simulink model "rtlsdr_datafm_ascii_audio"  (R2014b)
settings: Solver=ode45  StartTime=0.0  StopTime=60  RelTol=1e-3
PreLoadFcn:
  | %%%%%%%%%%%%%%%%%%%%%%%%%%%%%%%%%%%%%%%%%%%%%%%%%%%%%%%%%%%%%%%%%%%%%%%%%%%
  | % check to see if Simulink library folder is missing from the MATLAB path %
  | %%%%%%%%%%%%%%%%%%%%%%%%%%%%%%%%%%%%%%%%%%%%%%%%%%%%%%%%%%%%%%%%%%%%%%%%%%%
  | if isempty(strfind(path, 'rtlsdr_book_library'))
  | 
  |     % create error window
  |     fig_error = figure(...
  |         'Name', 'Error: RTL-SDR Book Library',...
  |         'Toolbar','none',...
  |         'MenuBar','none',...
  |         'NumberTitle','off',...
  |         'Resize','off',...
  |         'WindowStyle','modal');
  |     fig_error.Position(3) = 600;
  |     fig_error.Position(4) = 150;
  |     fig_axes = axes(...
  |         'Parent',fig_error,...
  |         'Position',[0,0,1,1],...
  |         'visible','off');
  |     % error message
  |     t_title = text(.05,.8,...
  |         'MISSING DIRECTORIES',...
  |         'FontSize',11.5);
  |     t_body = text(.075,.6,...
  |         [{'Simulink cannot find the  \it{<root>}\rm / \it{rtlsdr\_book\_library}\rm  folder in the \it{MATLAB Path}\rm.'},...
  |         {'Please set the MATLAB path following the instructions given in Exercise 2.4.'}],...
  |         'FontSize',10.5);
  |     % buttons
  |     btn_path = uicontrol(...
  |         'Parent',fig_error,...
  |         'String','Set Path Now',...
  |         'FontSize',10,...
  |         'Callback', 'pathtool; close(fig_error);',...
  |         'Position', [fig_error.Position(3)/2-210, 30, 200, 30]);
  |     btn_abort = uicontrol(...
  |         'Parent',fig_error,...
  |         'String','No thanks',...
  |         'FontSize',10,...
  |         'Callback', 'close(fig_error); abort=1;',...
  |         'Position', [fig_error.Position(3)/2+10, 30, 200, 30]);
  | 
  |     % pause to allow user to interact with error box
  |     uiwait(fig_error);
  | 
  |     % abort simulation
  |     try
  |         if abort==1
  |             set_param(gcs, 'SimulationCommand', 'stop');
  |         end
  |     end
  | 
  |     % if user has set path, allow diagram to be updated
  |     if ~exist('abort','var')
  |         % create error window
  |         fig_update = figure(...
  |             'Name', 'Update Diagram',...
  |             'Toolbar','none',...
  |             'MenuBar','none',...
  |             'NumberTitle','off',...
  |             'Resize','off');
  |         fig_update.Position(3) = 400;
  |         fig_update.Position(4) = 120;
  |         fig_axes = axes(...
  |             'Parent',fig_update,...
  |             'Position',[0,0,1,1],...
  |             'visible','off');
  |         % instruction message
  |         t_body = text(.075,.7,...
  |             'Once you have set the path, update the block diagram',...
  |             'FontSize',10.5);
  |         % button
  |         btn_update = uicontrol(...
  |             'Parent',fig_update,...
  |             'String','Update Block Diagram',...
  |             'FontSize',10,...
  |             'Callback', 'set_param(gcs,''SimulationCommand'',''update''); close(gcf)',...
  |             'Position', [fig_update.Position(3)/2-100, 30, 200, 30]);
  |     end
  | 
  |     % clear error components
  |     clear('fig_error','fig_update','fig_axes','t_title','t_body','btn_path','btn_abort','btn_update','abort');
  | 
  | end
  | %%%%%%%%%%%%%%%%%%%%%%%%%%%%%%%%%%%%%%%%%%%%%%%%%%%%%%%%%%%%%%%%%%%%%%%%%%%
undefined symbols (not defined in the file): dfilt, fdesignblkfcn, gcbh, rec, startfcn_spectrum_analyzer
libraries: simulink x5, dsparch4 x3, rtlsdr_book_library x3, dspmlti4 x2, commutil2 x2, commrfcorlib x1, dspstat3 x1, dspmtrx3 x1, sdrrlib x1, dspsnks4 x1
CloseFcn:
  | closefcn_model;
Description:
  | Software, Simulation Examples and Design Exercises Licence Agreement
  | 
  | This license agreement refers to the simulation examples, design exercises and files,
  | and associated software MATLAB and Simulink resources that accompany the book:
  | 
  |      Title: Software Defined Radio using MATLAB & Simulink and the RTL-SDR
  |      Published by Strathclyde Academic Media, 2015
  |      Authored by Robert W. Stewart, Kenneth W. Barlee, Dale S.W. Atkinson,
  |      and Louise H. Crockett
  | 
  | and made available as a download from, www.desktopSDR.com or variously acquired
  | by other means such as via USB storage, cloud storage, disk or any other electronic
  | or optical or magnetic storage mechanism. These files and associated software may
  | be used subject to the terms of agreement of the conditions below:
  | 
  |     Copyright © 2015 Robert W. Stewart, Kenneth W. Barlee, Dale S.W. Atkinson,
  |     and Louise H. Crockett
  |     All rights reserved.
  | 
  | Redistribution and use in source and binary forms, with or without modification, are
  | permitted provided that the following conditions are met:
  | 
  |    1.  Redistributions of source code must retain the above copyright notice, this list of
  |         conditions and the following disclaimer.
  | 
  |    2.  Redistributions in binary form must reproduce the above copyright notice, this
  |         list of conditions and the following disclaimer in the documentation and/or other
  |         materials provided with the distribution.
  | 
  |    3.  Neither the name of the copyright holder nor the names of its contributors may
  |         be used to endorse or promote products derived from this software without
  |         specific prior written permission.
  | 
  |    4.  In all cases, the software is, and all modifications and derivatives of the
  |         software shall be, licensed to you solely for use in conjunction with The
  |         MathWorks, Inc. products and service offerings.
  | 
  | THIS SOFTWARE IS PROVIDED BY THE COPYRIGHT HOLDERS AND CONTRIBUTORS
  | "AS IS" AND ANY EXPRESS OR IMPLIED WARRANTIES, INCLUDING, BUT NOT LIMITED
  | TO, THE IMPLIED WARRANTIES OF MERCHANTABILITY AND FITNESS FOR A
  | PARTICULAR PURPOSE ARE DISCLAIMED. IN NO EVENT SHALL THE COPYRIGHT
  | HOLDER OR CONTRIBUTORS BE LIABLE FOR ANY DIRECT, INDIRECT, INCIDENTAL,
  | SPECIAL, EXEMPLARY, OR CONSEQUENTIAL DAMAGES (INCLUDING, BUT NOT
  | LIMITED TO, PROCUREMENT OF SUBSTITUTE GOODS OR SERVICES; LOSS OF USE,
  | DATA, OR PROFITS; OR BUSINESS INTERRUPTION) HOWEVER CAUSED AND ON ANY
  | THEORY OF LIABILITY, WHETHER IN CONTRACT, STRICT LIABILITY, OR TORT
  | (INCLUDING NEGLIGENCE OR OTHERWISE) ARISING IN ANY WAY OUT OF THE USE
  | OF THIS SOFTWARE, EVEN IF ADVISED OF THE POSSIBILITY OF SUCH DAMAGE.
  | 
  | 
  | Audio Tracks used in Simulations Examples and Design Exercises
  | 
  | The music and vocal files used within the Examples files and software within the book
  | were variously written, arranged, performed, recorded and produced by Garrey Rice,
  | Adam Struth, Jamie Struth, Iain Thistlethwaite and also Marshall Craigmyle who
  | collectively, and individually where appropriate, assert and retain all of their copyright,
  | performance and artistic rights. Permission to use and reproduce this music is
  | granted for all purposes associated with MATLAB and Simulink software and the
  | simulation examples and design exercises files that accompany this book. Requests to
  | use the music for any other purpose should be directed to: info@desktopSDR.com.
  | For information on music track names, full credits, and links to the musicians please
  | refer to www.desktopSDR.com/more/audio.
settings Model: SimulationMode=accelerator  Creator=desktopSDR Team  LastModifiedBy=desktopSDR Team
settings DataIOCC: LimitDataPoints=off  SaveOutput=off  SignalLogging=off  SaveTime=off

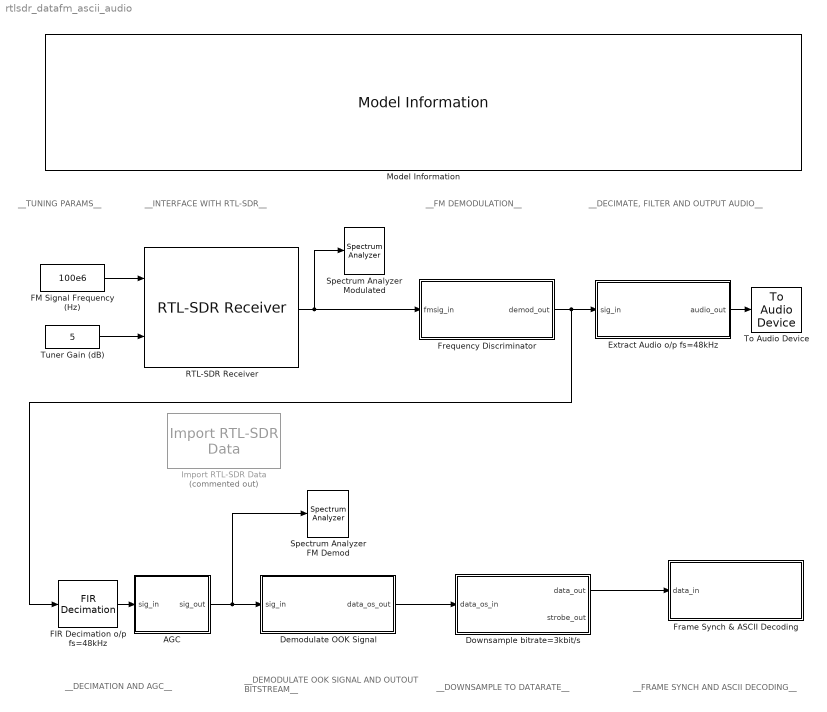
== system rtlsdr_datafm_ascii_audio ==
  note: __FRAME SYNCH AND ASCII DECODING__
  note: __DECIMATION AND AGC__
  note: __DOWNSAMPLE TO DATARATE__
  note: __DEMODULATE OOK SIGNAL
      | AND OUTOUT BITSTREAM__
  note: __FM DEMODULATION__
  note: __INTERFACE WITH RTL-SDR__
  note: __TUNING PARAMS__
  note: __DECIMATE, FILTER AND OUTPUT AUDIO__
  AGC : Subsystem
  Demodulate OOK Signal : Subsystem
  Downsample bitrate=3kbit/s : Subsystem  mask{fs=3e3}
      mask prompts: fs "Data bitrate (bit/s):"
      mask help: This block is used to downsample the received (oversampled) data back to its original bitrate. It comprises of an edge detector and a sampler.
  Extract Audio o/p fs=48kHz : Subsystem
  FIR Decimation o/p fs=48kHz : dspmlti4/FIR Decimation  h=firpm(150, [0 15e3 20e3 (240e3/2)]/(240e3/2), [1 1 0 0], [1 1],20)  D=5  filtStruct=Direct form  framing=Allow multirate processing  inputOffset=0  outputBufInitCond=0  InputProcessing=Columns as channels (frame based)  firstCoeffDataTypeStr=Inherit: Same word length as input  firstCoeffLastDataTypeStr=Inherit: Same word length as input  firstCoeffMin=[]  firstCoeffMax=[]  outputDataTypeStr=Inherit: Same as accumulator  outputLastDataTypeStr=Inherit: Same as accumulator  outputMin=[]  outputMax=[]  roundingMode=Floor  overflowMode=off  FilterSource=Specify via dialog  FilterObject=Hm_firdecim
      settings: allowOverrides=off
  "FM Signal Frequency (Hz) " : Constant  Value=100e6
  Frame Synch & ASCII Decoding : Subsystem  mask(Receiver Parameter Settings){msg_len=32, fs=3e3, ascii_len=8}
      mask prompts: msg_len "Message Length (chars)"; fs "Sampling Frequency"; ascii_len "ACSII Length"
      mask help: The subsystem implements frame synchronisation to re-frame the received data back to its original frame structure. The preamble is then removed before the payload data is ASCII decoded back to the transmitted string.
      mask Callback msg_len: ASCII_receive_mtchd_filt;
      mask Callback fs: ASCII_receive_mtchd_filt;
      mask Callback ascii_len: ASCII_receive_mtchd_filt;
  Frequency Discriminator : Subsystem
  Import RTL-SDR Data : rtlsdr_book_library/Additional Tools/Import RTL-SDR Data  Commented=on  filename=rec_data\datafm_ascii_audio.mat  frm_size=4096  data_type=single
  Model Information : rtlsdr_book_library/Additional Tools/Model Information/Model Information
  RTL-SDR Receiver : sdrrlib/RTL-SDR Receiver  SourceLibraryInfo="This block requires <a href=\"http://www.mathworks.com/hardware-support/rtl-sdr.html\">Communications System Toolbox Support Package for RTL-SDR Radio</a>"  sobjType=sdrr.internal.SDRRTLReceiverSL  IPAddress=0  dataUDPPort=-1  ctrlUDPPort=-1  subDeviceList=nosubdev  sdrBlockType=SDRBlockTypeSLT.SDRRxBlock  requester=UNUSED_BY_SFCN  sdrExecutionMode=SDRExecutionModeSLT.ExecModeHW  LostSamplesOutputPort=off  OutputDataType=single  FrameLength=4096  EnableBurstMode=off  NumFramesInBurst=20  BypassUserLogic=off  DecimatorSelect=DDC decimator  SourceSelect=RF data  SineAmplitude=16000  EnableInternalClock=off  BypassIQBalance=off  CenterFrequency=433.9e6  IFBandwidth=40e6  ADCRateSource=Dialog  ADCRate=240e3  CenterFrequencySource=Input port  GainSource=Input port  IntermediateFrequency=0  Gain=15  DecimationFactorSource=Dialog  DecimationFactor=512  RFFrequencyIsTunable=logical(1)  SampleTime=(4096)/(240e3)  IFBandwidthSource=Dialog  SineFrequency=30000  BypassDCBlockingFilter=off  IntermediateFrequencySource=Dialog  IQBalanceCoefficients=64  SkipAllHardwareResetAndInitialization=off  EnableIQCalibrationTable=on  CacheIQCalibrationTable=off  EnableOffsetTuning=off  EnableRTLAGC=off  EnableTestMode=off  EnableTunerAGC=off  FrequencyCorrectionSource=Dialog  FrequencyCorrection=0  NumMLBuffers=128  NumUSBBuffers=16  LatencyOutputPort=off  RTLCrystalFrequency=28800000  TunerCrystalFrequency=28800000
  Spectrum Analyzer FM Demod : SpectrumAnalyzer  StartFcn=startfcn_spectrum_analyzer;
  Spectrum Analyzer Modulated : SpectrumAnalyzer  StartFcn=startfcn_spectrum_analyzer;
  To Audio Device : dspsnks4/To Audio Device  deviceName=Default  inheritSampleRate=on  sampleRate=44100  deviceDatatype=Determine from input data type  autoBufferSize=on  bufferSize=4096  queueDuration=1.0  defaultOutputChannelMapping=on  outputChannelMapping=1:2  outputNumUnderrunSamples=off
  Tuner Gain (dB) : Constant  Value=5
  wires:
  Downsample bitrate=3kbit/s/1(data_out) -> Frame Synch & ASCII Decoding/1(data_in)
  FIR Decimation o/p fs=48kHz/1 -> AGC/1(sig_in)
  Tuner Gain (dB)/1 -> RTL-SDR Receiver/2
  "FM Signal Frequency (Hz) "/1 -> RTL-SDR Receiver/1
  Frequency Discriminator/1(demod_out) -> Extract Audio o/p fs=48kHz/1(sig_in), FIR Decimation o/p fs=48kHz/1
  Demodulate OOK Signal/1(data_os_out) -> Downsample bitrate=3kbit/s/1(data_os_in)
  AGC/1(sig_out) -> Demodulate OOK Signal/1(sig_in), Spectrum Analyzer FM Demod/1
  Extract Audio o/p fs=48kHz/1(audio_out) -> To Audio Device/1
  RTL-SDR Receiver/1 -> Spectrum Analyzer Modulated/1, Frequency Discriminator/1(fmsig_in)

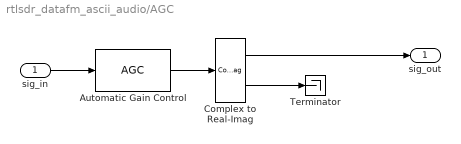
== system rtlsdr_datafm_ascii_audio/AGC ==
  sig_in : Inport
  Automatic Gain Control : commrfcorlib/AGC  SimulateUsing=Code generation  DetectorMethod=Rectifier  LoopMethod=Linear  UpdatePeriod=128  StepSize=0.03  MaximumGain=20  GainOutputPort=off
  Complex to Real-Imag : ComplexToRealImag
  Terminator : Terminator
  sig_out : Outport
  wires:
  Complex to Real-Imag/1 -> sig_out/1
  Automatic Gain Control/1 -> Complex to Real-Imag/1
  sig_in/1 -> Automatic Gain Control/1
  Complex to Real-Imag/2 -> Terminator/1

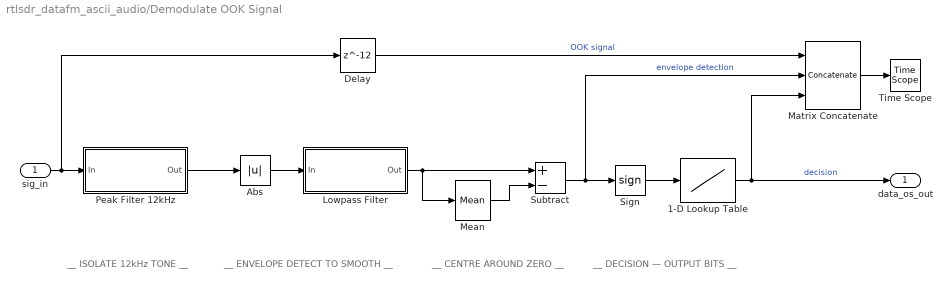
== system rtlsdr_datafm_ascii_audio/Demodulate OOK Signal ==
  note: __ ISOLATE 12kHz TONE __
  note: __ ENVELOPE DETECT TO SMOOTH __
  note: __ CENTRE AROUND ZERO __
  note: __ DECISION — OUTPUT BITS __
  sig_in : Inport
  1-D Lookup Table : Lookup_n-D  NumberOfTableDimensions=1  BreakpointsForDimension1=[-1,0,1]  Table=[0,0,1]  InternalRulePriority=Speed  RndMeth=Simplest  InputSameDT=on
  Abs : Abs
  Delay : Delay  DelayLength=12  InputProcessing=Columns as channels (frame based)
  Lowpass Filter : Subsystem  DialogController=fdesignblkfcn  InitFcn=fdesignblkfcn(gcbh, {'InitFcn'});  mask(Lowpass Filter){}
      mask help: Design a lowpass filter
      settings: CopyFcn=fdesignblkfcn(gcbh, {'CopyFcn'});
      mask Help: helpview(mapfilelocation('dsp'), 'dsplowpassfilter');
      mask Display: disp('Lowpass')
  Matrix Concatenate : Concatenate  NumInputs=3  Mode=Multidimensional array  ConcatenateDimension=2
  Mean : dspstat3/Mean  run=off  reset_popup=None  InputProcessing=Columns as channels (frame based)  directionMode=Each column  dimension=1  treatSBRowAsCol=on  roiEnable=off  roiType=Rectangles  roiPortion=Entire ROI  roiOutput=Individual statistics for each ROI  roiFlag=off  outputDataTypeStr=Inherit: Same as accumulator  outputLastDataTypeStr=Inherit: Same as accumulator  outputMin=[]  outputMax=[]  roundingMode=Floor  overflowMode=off
  Peak Filter 12kHz : Subsystem  DialogController=fdesignblkfcn  InitFcn=fdesignblkfcn(gcbh, {'InitFcn'});  mask(Peak/Notch Filter){}
      mask help: Design a peak/notch filter
      settings: CopyFcn=fdesignblkfcn(gcbh, {'CopyFcn'});
      mask Help: helpview(mapfilelocation('dsp'), 'dsppeaknotchfilter');
      mask Display: disp('Peak-Notch');
  Sign : Signum
  Subtract : Sum  Inputs=+-
  Time Scope : TimeScope  StartFcn=startfcn_time_scope  DefaultConfigurationName=spbscopes.TimeScopeBlockCfg
  data_os_out : Outport
  wires:
  Abs/1 -> Lowpass Filter/1(In)
  Lowpass Filter/1(Out) -> Subtract/1, Mean/1
  Peak Filter 12kHz/1(Out) -> Abs/1
  Sign/1 -> 1-D Lookup Table/1
  1-D Lookup Table/1 -> Matrix Concatenate/3, data_os_out/1  "decision"
  Subtract/1 -> Matrix Concatenate/2, Sign/1  "envelope detection"
  Mean/1 -> Subtract/2
  sig_in/1 -> Peak Filter 12kHz/1(In), Delay/1
  Matrix Concatenate/1 -> Time Scope/1
  Delay/1 -> Matrix Concatenate/1  "OOK signal"

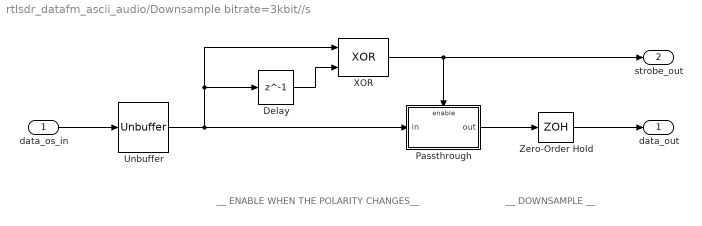
== system rtlsdr_datafm_ascii_audio/Downsample bitrate=3kbit//s ==
  note: __ DOWNSAMPLE __
  note: __ ENABLE WHEN THE POLARITY CHANGES__
  data_os_in : Inport
  Delay : Delay  DelayLength=1  InitialCondition=0
  Passthrough : Subsystem
  Unbuffer : Unbuffer  SampleBasedProcessing=Same as frame based
  XOR : Logic  Operator=XOR  IconShape=distinctive  AllPortsSameDT=off  OutDataTypeStr=boolean
  Zero-Order Hold : ZeroOrderHold  SampleTime=1/fs
  data_out : Outport
  strobe_out : Outport  Port=2
  wires:
  Zero-Order Hold/1 -> data_out/1
  Unbuffer/1 -> Delay/1, XOR/1, Passthrough/1(in)
  Delay/1 -> XOR/2
  XOR/1 -> strobe_out/1, Passthrough/Enable
  Passthrough/1(out) -> Zero-Order Hold/1
  data_os_in/1 -> Unbuffer/1

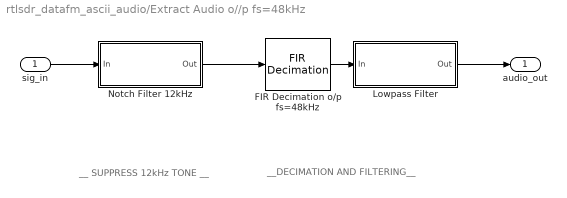
== system rtlsdr_datafm_ascii_audio/Extract Audio o//p fs=48kHz ==
  note: __ SUPPRESS 12kHz TONE __
  note: __DECIMATION AND FILTERING__
  sig_in : Inport
  FIR Decimation o/p fs=48kHz : dspmlti4/FIR Decimation  h=firpm(150, [0 15e3 20e3 (240e3/2)]/(240e3/2), [1 1 0 0], [1 1],20)  D=5  filtStruct=Direct form  framing=Allow multirate processing  inputOffset=0  outputBufInitCond=0  InputProcessing=Columns as channels (frame based)  firstCoeffDataTypeStr=Inherit: Same word length as input  firstCoeffLastDataTypeStr=Inherit: Same word length as input  firstCoeffMin=[]  firstCoeffMax=[]  outputDataTypeStr=Inherit: Same as accumulator  outputLastDataTypeStr=Inherit: Same as accumulator  outputMin=[]  outputMax=[]  roundingMode=Floor  overflowMode=off  FilterSource=Specify via dialog  FilterObject=Hm_firdecim
      settings: allowOverrides=off
  Lowpass Filter : Subsystem  DialogController=fdesignblkfcn  InitFcn=fdesignblkfcn(gcbh, {'InitFcn'});  mask(Lowpass Filter){}
      mask help: Design a lowpass filter
      settings: CopyFcn=fdesignblkfcn(gcbh, {'CopyFcn'});
      mask Help: helpview(mapfilelocation('dsp'), 'dsplowpassfilter');
      mask Display: disp('Lowpass')
  Notch Filter 12kHz : Subsystem  DialogController=fdesignblkfcn  InitFcn=fdesignblkfcn(gcbh, {'InitFcn'});  mask(Peak/Notch Filter){}
      mask help: Design a peak/notch filter
      settings: CopyFcn=fdesignblkfcn(gcbh, {'CopyFcn'});
      mask Help: helpview(mapfilelocation('dsp'), 'dsppeaknotchfilter');
      mask Display: disp('Peak-Notch');
  audio_out : Outport
  wires:
  Notch Filter 12kHz/1(Out) -> FIR Decimation o/p fs=48kHz/1
  sig_in/1 -> Notch Filter 12kHz/1(In)
  FIR Decimation o/p fs=48kHz/1 -> Lowpass Filter/1(In)
  Lowpass Filter/1(Out) -> audio_out/1

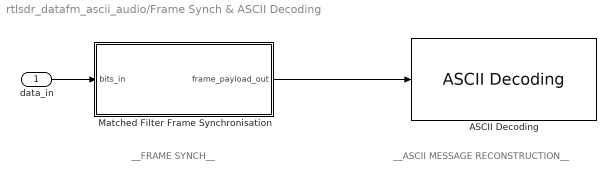
== system rtlsdr_datafm_ascii_audio/Frame Synch & ASCII Decoding ==
  note: __FRAME SYNCH__
  note: __ASCII MESSAGE RECONSTRUCTION__
  data_in : Inport
  ASCII Decoding : rtlsdr_book_library/Data Comms Sources and Sinks/ASCII Decoding  msg_len=msg_len  ascii_len=ascii_len
  Matched Filter Frame Synchronisation : Subsystem
  wires:
  data_in/1 -> Matched Filter Frame Synchronisation/1(bits_in)
  Matched Filter Frame Synchronisation/1(frame_payload_out) -> ASCII Decoding/1

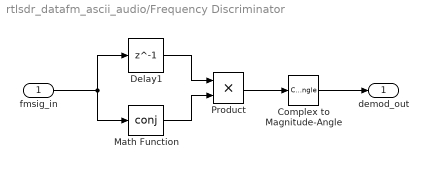
== system rtlsdr_datafm_ascii_audio/Frequency Discriminator ==
  fmsig_in : Inport
  Complex to Magnitude-Angle : ComplexToMagnitudeAngle  Output=Angle
  Delay1 : Delay  DelayLength=1  InitialCondition=0  InputProcessing=Columns as channels (frame based)
  Math Function : Math  Operator=conj  SaturateOnIntegerOverflow=on
  Product : Product
  demod_out : Outport
  wires:
  fmsig_in/1 -> Delay1/1, Math Function/1
  Delay1/1 -> Product/1
  Product/1 -> Complex to Magnitude-Angle/1
  Math Function/1 -> Product/2
  Complex to Magnitude-Angle/1 -> demod_out/1

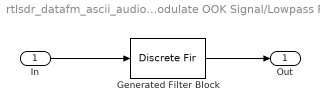
== system rtlsdr_datafm_ascii_audio/Demodulate OOK Signal/Lowpass Filter ==
  In : Inport
  Generated Filter Block : DiscreteFir  Tag=BlockMethodSubSystem  Coefficients=[-0.056889882382706855 0.04272587047701297 0.041865722441748722 0.046827868588471426 0.055061875523844783 0.064544738333393775 0.073956118454246697 0.082302711912541626 0.088820221635909913 0.092955621228906521 0.094371888653913771 0.092955621228906521 0.088820221635909913 0.082302711912541626 0.073956118454246697 0.064544738333393775 0.055061875523844783 0.046827868588471426 0.041865722441748722 0.04272587047701297 -0.056889882382706855]  InputProcessing=Columns as channels (frame based)
  Out : Outport
  wires:
  Generated Filter Block/1 -> Out/1
  In/1 -> Generated Filter Block/1

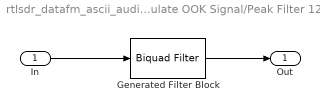
== system rtlsdr_datafm_ascii_audio/Demodulate OOK Signal/Peak Filter 12kHz ==
  In : Inport
  Generated Filter Block : dsparch4/Biquad Filter  Tag=BlockMethodSubSystem  IIRFiltStruct=Direct form II  CoeffSource=Specify via dialog  BiQuadCoeffs=[0.5 0 -0.5 1 0 0.66817863791929899]  a0Flag=Warning  IC=0  ICnum=0  ICden=0  InputProcessing=Columns as channels (frame based)  denAccumFracLength=30  denProdOutputFracLength=30  secondMemoryFracLength=15  roundingMode=Floor  overflowMode=off  ScaleValues=[0.33182136208070101;1]  optimizeScaleValues=off  ScaleValueMode=Specify via input port (g)  scaleValueFracLength=14  FilterSource=Specify via dialog  dfiltObjectName=dfilt.df2tsos([1 0.3 0.4],[1 0.1 0.2])
  Out : Outport
  wires:
  In/1 -> Generated Filter Block/1
  Generated Filter Block/1 -> Out/1

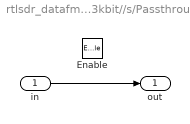
== system rtlsdr_datafm_ascii_audio/Downsample bitrate=3kbit//s/Passthrough ==
  in : Inport
  Enable : EnablePort
  out : Outport
  wires:
  in/1 -> out/1

== system rtlsdr_datafm_ascii_audio/Extract Audio o//p fs=48kHz/Lowpass Filter ==
  In : Inport
  Generated Filter Block : dsparch4/Biquad Filter  Tag=BlockMethodSubSystem  IIRFiltStruct=Direct form II  CoeffSource=Specify via dialog  BiQuadCoeffs=[0.042969561565618077 0.085939123131236153 0.042969561565618077 1 -1.555657758639478 0.87862894950711246;0.061935778665187145 0.12387155733037429 0.061935778665187145 1 -1.4205854439157277 0.71551417743867618;0.076267506257963871 0.15253501251592774 0.076267506257963871 1 -1.3129466799361755 0.58552845469333503;0.086601072542009133 0.17320214508401827 0.086601072542009133 1 -1.2285300304649582 0.48358600582481348;0.093330556989539987 0.18666111397907997 0.093330556989539987 1 -1.163928907888546 0.40557299919227274;0.096444753467057845 0.19288950693411569 0.096444753467057845 1 -1.1165183760349042 0.34831953379659664;0.093941235402774201 0.1878824708055484 0.093941235402774201 1 -1.0843804969696778 0.30950948727293498;0.06178520401543218 0.12357040803086436 0.06178520401543218 1 -1.0662257647565232 0.28758563845929269;0.055723392794766298 0.1114467855895326 0.055723392794766298 1 -1.0621451972418323 0.28265790148054942;0.057022086237706486 0.11404417247541297 0.057022086237706486 1 -1.0736131368995174 0.29650670807858259;0.059076157735379158 0.11815231547075832 0.059076157735379158 1 -1.0986348427077246 0.32672318765855057;0.061968373960671889 0.12393674792134378 0.061968373960671889 1 -1.1382102890943879 0.37451492003590464;0.065816095114757556 0.13163219022951511 0.065816095114757556 1 -1.1939341274770339 0.44180762331972157;0.070775447994568252 0.1415508959891365 0.070775447994568252 1 -1.2680675169023181 0.53133189736134834;0.077044306786640995 0.15408861357328199 0.077044306786640995 1 -1.3636185258276994 0.64672031780597239;0.027416633436479335 0.054833266872958669 0.027416633436479335 1 -1.4843995625697666 0.79257678971633061;0.025182438141471038 0.050364876282942075 0.025182438141471038 1 -1.6349915970637752 0.97443334138682025;0.04855389746467715 0.097107794929354299 0.04855389746467715 1 -1.5190593292115486 0.83443229465294233;0.067085454415403187 0.13417090883080637 0.067085454415403187 1 -1.3912817200511742 0.68012668705103563;0.081497123248148048 0.1629942464962961 0.081497123248148048 1 -1.2898124076148489 0.55759125998115422;0.092395363974827269 0.18479072794965454 0.092395363974827269 1 -1.210637439466447 0.46197872154598202;0.10020909151780877 0.20041818303561754 0.10020909151780877 1 -1.1505510212366299 0.38941772017415877;0.10527662371649776 0.21055324743299553 0.10527662371649776 1 -1.1071126518721077 0.33696108068878605;0.10764709070254799 0.21529418140509599 0.10764709070254799 1 -1.0785684378951543 0.30249078256554834;0.061743519146292225 0.12348703829258445 0.061743519146292225 1 -1.0637754129904147 0.28462656745622505;0.055510029644634425 0.11102005928926885 0.055510029644634425 1 -1.061331093635125 0.28167478125698797;0.056629126444816269 0.11325825288963254 0.056629126444816269 1 -1.0695023053542168 0.29154242393275437;0.058487856243194969 0.11697571248638994 0.058487856243194969 1 -1.0910637531749297 0.31758025895419473;0.06116095659595399 0.12232191319190798 0.06116095659595399 1 -1.1268755842462319 0.36082700921901179;0.064756747550877514 0.12951349510175503 0.064756747550877514 1 -1.1783777543589316 0.42302158074274743;0.069421296340545946 0.13884259268109189 0.069421296340545946 1 -1.2476572474610272 0.50668423766453741;0.075341935222395684 0.15068387044479137 0.075341935222395684 1 -1.3375283160935707 0.61521350145575437;0.076281548564130483 0.15256309712826097 0.076281548564130483 1 -1.4516002590171362 0.75296799990671892;0.27118984696313492 0.54237969392626983 0.27118984696313492 1 -1.5942748095188128 0.92526331321828925]  a0Flag=Warning  IC=0  ICnum=0  ICden=0  InputProcessing=Columns as channels (frame based)  denAccumFracLength=30  denProdOutputFracLength=30  secondMemoryFracLength=15  roundingMode=Floor  overflowMode=off  ScaleValues=[0.067729897263719196;1;1;1;1;1;1;1;1;1;1;1;1;1;1;1;1;1;1;1;1;1;1;1;1;1;1;1;1;1;1;1;1;1;1]  optimizeScaleValues=off  ScaleValueMode=Specify via input port (g)  scaleValueFracLength=14  FilterSource=Specify via dialog  dfiltObjectName=dfilt.df2tsos([1 0.3 0.4],[1 0.1 0.2])
  Out : Outport
  wires:
  Generated Filter Block/1 -> Out/1
  In/1 -> Generated Filter Block/1

== system rtlsdr_datafm_ascii_audio/Extract Audio o//p fs=48kHz/Notch Filter 12kHz ==
  In : Inport
  Generated Filter Block : dsparch4/Biquad Filter  Tag=BlockMethodSubSystem  IIRFiltStruct=Direct form II  CoeffSource=Specify via dialog  BiQuadCoeffs=[1.051462288938775 -2 1.05146208976721 1 -1.8906743662652825 0.98217615847856421;1.0514623541957084 -2 1.0514621640514155 1 -1.878343671696399 0.98114068021814849]  a0Flag=Warning  IC=0  ICnum=0  ICden=0  InputProcessing=Columns as channels (frame based)  denAccumFracLength=30  denProdOutputFracLength=30  secondMemoryFracLength=15  roundingMode=Floor  overflowMode=off  ScaleValues=[0.0053510810621176137;1;165.93249752671582]  optimizeScaleValues=off  ScaleValueMode=Specify via input port (g)  scaleValueFracLength=14  FilterSource=Specify via dialog  dfiltObjectName=dfilt.df2tsos([1 0.3 0.4],[1 0.1 0.2])
  Out : Outport
  wires:
  Generated Filter Block/1 -> Out/1
  In/1 -> Generated Filter Block/1

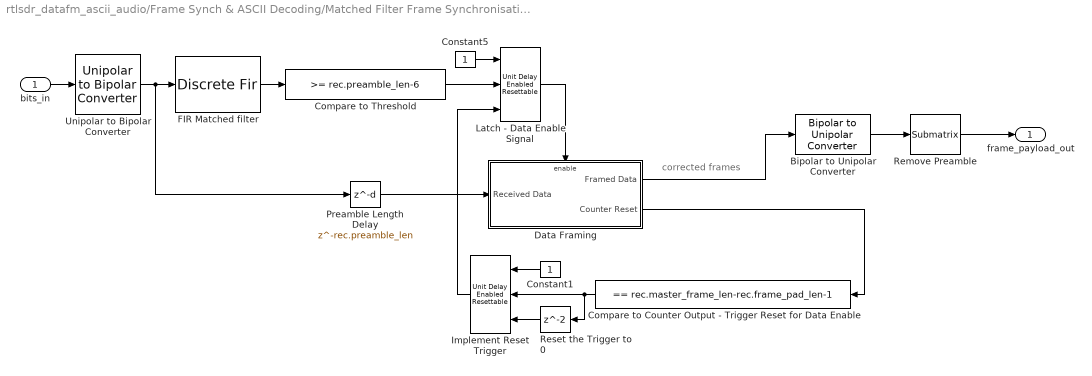
== system rtlsdr_datafm_ascii_audio/Frame Synch & ASCII Decoding/Matched Filter Frame Synchronisation ==
  note: corrected frames
  bits_in : Inport
  Bipolar to Unipolar Converter : commutil2/Bipolar to Unipolar Converter  M=2  polarity=Positive  dataType=Inherit via internal rule
  Compare to Counter Output - Trigger Reset for Data Enable : simulink/Logic and Bit Operations/Compare To Constant  relop===  const=rec.master_frame_len-rec.frame_pad_len-1  OutDataTypeStr=boolean
  Compare to Threshold : simulink/Logic and Bit Operations/Compare To Constant  relop=>=  const=rec.preamble_len-6  OutDataTypeStr=boolean
  Constant1 : Constant
  Constant5 : Constant
  Data Framing : Subsystem
  FIR Matched filter : DiscreteFir  Coefficients=rec.filter_coeff  InputProcessing=Columns as channels (frame based)
  Implement Reset Trigger : simulink/Additional Math & Discrete/Additional Discrete/Unit Delay Enabled Resettable  vinit=0  tsamp=-1
  Latch - Data Enable Signal : simulink/Additional Math & Discrete/Additional Discrete/Unit Delay Enabled Resettable  vinit=0  tsamp=-1
  Preamble Length Delay : Delay  DelayLength=rec.preamble_len  DelayLengthUpperLimit=10000  InitialCondition=1
  Remove Preamble : dspmtrx3/Submatrix  RowSpan=Range of rows  RowStartMode=Index  RowStartIndex=rec.preamble_len+rec.preamble_pad_len+1  RowEndMode=Index  RowEndIndex=rec.master_frame_len-rec.frame_pad_len  ColSpan=One column  ColStartMode=First  ColStartIndex=1  ColEndMode=Last  ColEndIndex=1
  Reset the Trigger to 0 : Delay  DelayLengthUpperLimit=10000  InitialCondition=0
  Unipolar to Bipolar Converter : commutil2/Unipolar to Bipolar Converter  M=2  polarity=Positive  dataType=Inherit via internal rule
  frame_payload_out : Outport
  wires:
  Unipolar to Bipolar Converter/1 -> FIR Matched filter/1, Preamble Length Delay/1
  Bipolar to Unipolar Converter/1 -> Remove Preamble/1
  Data Framing/2(Counter Reset) -> Compare to Counter Output - Trigger Reset for Data Enable/1
  Reset the Trigger to 0/1 -> Implement Reset Trigger/3
  FIR Matched filter/1 -> Compare to Threshold/1
  Preamble Length Delay/1 -> Data Framing/1(Received Data)
  Data Framing/1(Framed Data) -> Bipolar to Unipolar Converter/1
  Compare to Counter Output - Trigger Reset for Data Enable/1 -> Implement Reset Trigger/2, Reset the Trigger to 0/1
  Compare to Threshold/1 -> Latch - Data Enable Signal/2
  Constant1/1 -> Implement Reset Trigger/1
  bits_in/1 -> Unipolar to Bipolar Converter/1
  Constant5/1 -> Latch - Data Enable Signal/1
  Implement Reset Trigger/1 -> Latch - Data Enable Signal/3
  Remove Preamble/1 -> frame_payload_out/1
  Latch - Data Enable Signal/1 -> Data Framing/Enable

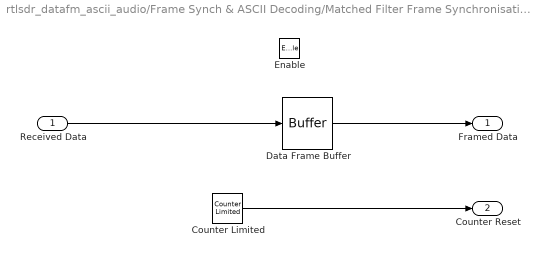
== system rtlsdr_datafm_ascii_audio/Frame Synch & ASCII Decoding/Matched Filter Frame Synchronisation/Data Framing ==
  Received Data : Inport
  Enable : EnablePort
  Counter Limited : simulink/Sources/Counter Limited  uplimit=rec.master_frame_len-rec.frame_pad_len-1  tsamp=-1
  Data Frame Buffer : Buffer  N=rec.master_frame_len-rec.frame_pad_len  TreatMby1Signals=One channel
  Framed Data : Outport
  Counter Reset : Outport  Port=2
  wires:
  Received Data/1 -> Data Frame Buffer/1
  Data Frame Buffer/1 -> Framed Data/1
  Counter Limited/1 -> Counter Reset/1
